simulink model "Telecom_PPM"  (R2015a)
settings: Solver=ode45  StartTime=0.0  StopTime=1000.0  RelTol=1e-3
libraries: simulink x1
settings Model: Creator=klkou  LastModifiedBy=klkou

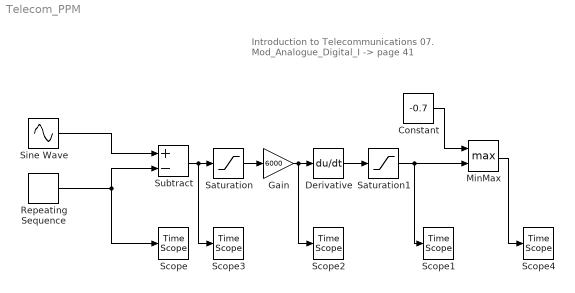
== system Telecom_PPM ==
  note: Introduction to Telecommunications
      | 07. Mod_Analogue_Digital_I -> page 41
  Constant : Constant  Value=-0.7
  Derivative : Derivative
  Gain : Gain  Gain=6000
  MinMax : MinMax  Function=max  Inputs=2
  Repeating Sequence : simulink/Sources/Repeating Sequence  rep_seq_t=[0 25]  rep_seq_y=[-2 2]
  Saturation : Saturate  UpperLimit=0.0005  LowerLimit=-0.0005
  Saturation1 : Saturate  UpperLimit=3  LowerLimit=-3
  Scope{,1..4} (5 alike) : TimeScope
  Sine Wave : Sin  Frequency=0.01  SampleTime=0
  Subtract : Sum  Inputs=+-
  wires:
  Repeating Sequence/1 -> Subtract/2, Scope/1
  Sine Wave/1 -> Subtract/1
  Derivative/1 -> Saturation1/1
  Saturation/1 -> Gain/1
  Subtract/1 -> Scope3/1, Saturation/1
  Gain/1 -> Scope2/1, Derivative/1
  Saturation1/1 -> MinMax/2, Scope1/1
  Constant/1 -> MinMax/1
  MinMax/1 -> Scope4/1
